simulink model "example_House_RoomFloorHeating"  (R2013b)
settings: Solver=ode23tb  StartTime=0.0  StopTime=24*3600  RelTol=1e-3
libraries: carnot x8
settings Model: Creator=drhf  LastModifiedBy=drhf
settings OptimizationCC: ExpressionDepthLimit=2147483647
settings DebuggingCC: StateNameClashWarn=warning
settings GRTTargetCC: CombineOutputUpdateFcns=off  GRTInterface=on

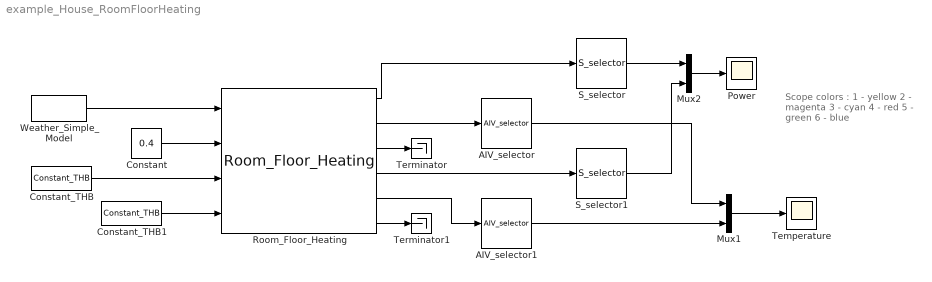
== system example_House_RoomFloorHeating ==
  note: Scope colors :
      | 1 - yellow
      | 2 - magenta
      | 3 - cyan
      | 4 - red
      | 5 - green
      | 6 - blue
  AIV_selector : carnot/Outputs/AIV_selector  e1=on  e2=on  e3=on  e4=off  e5=off  e6=off  e7=off  e8=off  e9=off
  AIV_selector1 : carnot/Outputs/AIV_selector  e1=on  e2=on  e3=on  e4=off  e5=off  e6=off  e7=off  e8=off  e9=off
  Constant : Constant  Value=0.4
  Constant_THB : carnot/Source/Simple/Constant_THB  t=22  mdot=600/3600  p=1e5  mID=No Pressure Drop  fluid=Water  mix=0  mix2=0  mix3=0  dia=0.02  hgt=0
  Constant_THB1 : carnot/Source/Simple/Constant_THB  t=30  mdot=600/3600  p=1e5  mID=No Pressure Drop  fluid=Water  mix=0  mix2=0  mix3=0  dia=0.02  hgt=0
  Mux1 : Mux  Inputs=2
  Mux2 : Mux  Inputs=2
  Power : Scope
      settings: YMin=0  YMax=12
  Room_Floor_Heating : carnot/Load/Houses/Room_Floor_Heating  t0=20  temp_neighbour=20
  S_selector : carnot/Outputs/S_selector  e1=off  e2=off  e3=off  e4=off  e5=off  e6=off  e7=on  e8=on  e9=off  e10=off  e11=off  e12=off  e13=off
  S_selector1 : carnot/Outputs/S_selector  e1=off  e2=off  e3=off  e4=off  e5=off  e6=off  e7=on  e8=on  e9=off  e10=off  e11=off  e12=off  e13=off
  Temperature : Scope
  Terminator : Terminator
  Terminator1 : Terminator
  Weather_Simple_Model : carnot/Weather/Weather_Simple_Model  lat=60  Ibn=900  Idg=100  tamb=5  deltaTsky=-6  rh=50  precip="10e-3/24/3600           % 10 mm in 24 h"  cloud=0.125  p=1013e2  vw=1  wdir=270
  wires:
  Weather_Simple_Model/1 -> Room_Floor_Heating/1
  Constant/1 -> Room_Floor_Heating/2
  Constant_THB/1 -> Room_Floor_Heating/3
  Constant_THB1/1 -> Room_Floor_Heating/4
  Room_Floor_Heating/1 -> S_selector/1
  Room_Floor_Heating/2 -> AIV_selector/1
  Room_Floor_Heating/5 -> AIV_selector1/1
  Room_Floor_Heating/4 -> S_selector1/1
  Room_Floor_Heating/3 -> Terminator/1
  Room_Floor_Heating/6 -> Terminator1/1
  Mux1/1 -> Temperature/1
  AIV_selector/1 -> Mux1/1
  AIV_selector1/1 -> Mux1/2
  S_selector/1 -> Mux2/1
  S_selector1/1 -> Mux2/2
  Mux2/1 -> Power/1
